simulink model "top_model_rw_desatTest"  (R2017b)
settings: Solver=FixedStepAuto  StartTime=0.0  StopTime=30000  FixedStep=.2  RelTol=1e-3  EnableMultiTasking=on
model workspace: external: MATLAB File C:\Users\Justin\Documents\00 MEng Project\PAN_ADCS\initialization\simulink_workspace_init.m (data not in the file)
undefined symbols (not defined in the file): h_init, hdmax, hmax, IAU, Imp_max, Imp_min, init, K_F, Kd, km, Kp, L_F, m_follower, match_tol, muE, ontime_max, ontime_min, q_init, s, Thrust_max, Thrust_min, wbn_init
libraries: aerolibtransform2 x12, aerolibconvert2 x8, sharedtransform x8, hEemethod x8, aerolibgravity2 x6, aerolibutil x6, aerolibcelestial x4, vrlib x4
(part 2 of 5)

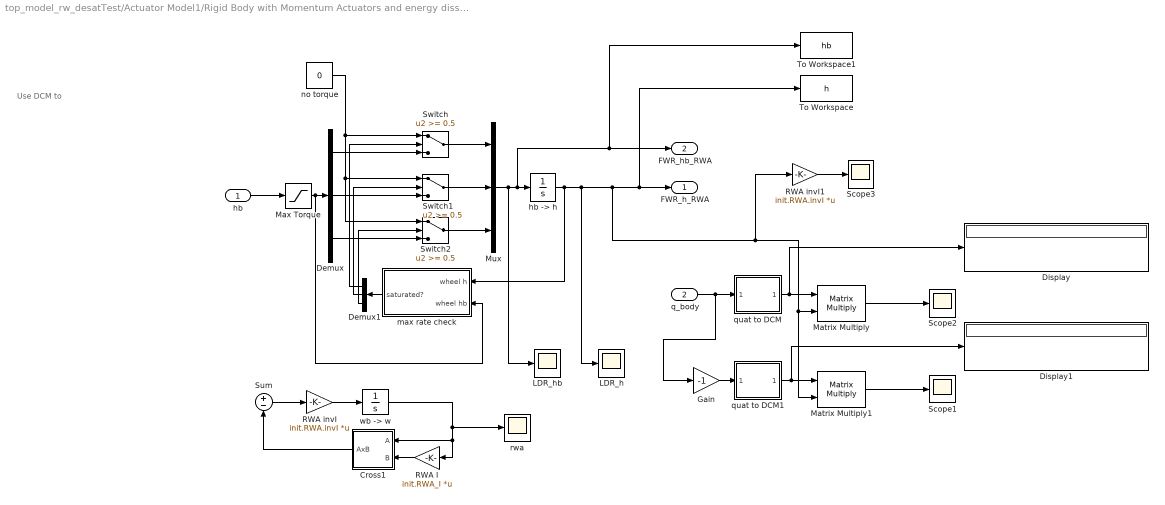
== system top_model_rw_desatTest/Actuator Model1/Rigid Body with Momentum Actuators and energy dissipation ==
  note: Use DCM to
  hb : Inport
  q_body : Inport  Port=2
  Cross1 : Subsystem
  Demux : Demux  Outputs=3
  Demux1 : Demux  Outputs=3
  Display : Display
  Display1 : Display
  Gain : Gain  Gain=-1
  LDR_h : Scope
  LDR_hb : Scope
  Matrix Multiply : Product  Multiplication=Matrix(*)
  Matrix Multiply1 : Product  Multiplication=Matrix(*)
  Max Torque : Saturate  UpperLimit=init.hdmax  LowerLimit=-init.hdmax
  Mux : Mux  Inputs=3
  RWA I : Gain  Gain=init.RWA_I  Multiplication=Matrix(K*u)
  RWA invI : Gain  Gain=init.RWA.invI  Multiplication=Matrix(K*u)
  RWA invI1 : Gain  Gain=init.RWA.invI  Multiplication=Matrix(K*u)
  Scope1 : Scope
  Scope2 : Scope
  Scope3 : Scope
  Sum : Sum  Inputs=+|-
  Switch : Switch  Threshold=0.5  SaturateOnIntegerOverflow=on  InputSameDT=on
  Switch1 : Switch  Threshold=0.5  SaturateOnIntegerOverflow=on  InputSameDT=on
  Switch2 : Switch  Threshold=0.5  SaturateOnIntegerOverflow=on  InputSameDT=on
  To Workspace : ToWorkspace  VariableName=h  SaveFormat=Timeseries  SampleTime=-1
  To Workspace1 : ToWorkspace  VariableName=hb  SaveFormat=Timeseries  SampleTime=-1
  "hb -> h" : Integrator  InitialCondition=init.FWR.h
  max rate check : Subsystem
  no torque : Constant  Value=0
  quat to DCM : Subsystem  mask(Direction Cosine Matrix){}
      mask help: Determines the 3x3 Direction Cosine Matrix (DCM) from a 4x1 quaternion orientation vector. The outputted DCM transforms vectors from inertial axes to body axes. This version corrects the fucked-up MATLAB one.
      mask Help:
      | <p>This block determines the 3x3 Direction Cosine Matrix (DCM) from a 4x1 quaternion orientation vector. The outputted DCM transforms vectors from inertial axes to body axes.  This version corrects the fucked-up MATLAB one</p>
      | 
      | <p>The block input and output contain more than one signal as described below.</p>
      | 
      | <p><H4>Block Vector Input - Quaternion</H4>
      | <ul>
      | <li>q0</li>
      | <li>q1</li>
      | <li>q2</li>
      | <li>q3</li>
      | </ul>
      | </p>
      | 
      | <p><H4>Block Matrix Output - Direction Cosine Matrix  </H4>
      |     <ul>
      |    </ul>
      |    </p>
      mask Display: disp('q to Q')
  quat to DCM1 : Subsystem  mask(Direction Cosine Matrix){}
      mask help: Determines the 3x3 Direction Cosine Matrix (DCM) from a 4x1 quaternion orientation vector. The outputted DCM transforms vectors from inertial axes to body axes. This version corrects the fucked-up MATLAB one.
      mask Help:
      | <p>This block determines the 3x3 Direction Cosine Matrix (DCM) from a 4x1 quaternion orientation vector. The outputted DCM transforms vectors from inertial axes to body axes.  This version corrects the fucked-up MATLAB one</p>
      | 
      | <p>The block input and output contain more than one signal as described below.</p>
      | 
      | <p><H4>Block Vector Input - Quaternion</H4>
      | <ul>
      | <li>q0</li>
      | <li>q1</li>
      | <li>q2</li>
      | <li>q3</li>
      | </ul>
      | </p>
      | 
      | <p><H4>Block Matrix Output - Direction Cosine Matrix  </H4>
      |     <ul>
      |    </ul>
      |    </p>
      mask Display: disp('q to Q')
  rwa : Scope
  "wb -> w" : Integrator  InitialCondition=[0;0;0]
  FWR_h_RWA : Outport
  FWR_hb_RWA : Outport  Port=2
  wires:
  hb/1 -> Max Torque/1
  Mux/1 -> To Workspace1/1, FWR_hb_RWA/1, "hb -> h"/1, LDR_hb/1
  Max Torque/1 -> Demux/1, max rate check/2(wheel hb)
  max rate check/1(saturated?) -> Demux1/1
  Demux1/1 -> Switch/2
  Demux1/2 -> Switch1/2
  Demux1/3 -> Switch2/2
  no torque/1 -> Switch/1, Switch1/1, Switch2/1
  Demux/1 -> Switch/3
  Demux/2 -> Switch1/3
  Demux/3 -> Switch2/3
  Switch/1 -> Mux/1
  Switch1/1 -> Mux/2
  Switch2/1 -> Mux/3
  q_body/1 -> Gain/1, quat to DCM/1(e0 e1 e2 e3)
  quat to DCM/1(DCM) -> Display/1, Matrix Multiply/1
  Matrix Multiply/1 -> Scope2/1
  Matrix Multiply1/1 -> Scope1/1
  quat to DCM1/1(DCM) -> Display1/1, Matrix Multiply1/1
  "hb -> h"/1 -> max rate check/1(wheel h), RWA invI1/1, Matrix Multiply1/2, Matrix Multiply/2, To Workspace/1, FWR_h_RWA/1, LDR_h/1
  Gain/1 -> quat to DCM1/1(e0 e1 e2 e3)
  RWA I/1 -> Cross1/2(B)
  "wb -> w"/1 -> rwa/1, Cross1/1(A), RWA I/1
  Cross1/1(AxB) -> Sum/2
  Sum/1 -> RWA invI/1
  RWA invI/1 -> "wb -> w"/1
  RWA invI1/1 -> Scope3/1
  ? -> Sum/1

== system top_model_rw_desatTest/Actuator Model1/torque_mt ==
  A : Inport
  B : Inport  Port=2
  Mux4 : Mux  Inputs=3
  Product{,1..5} (6 alike) : Product  SaturateOnIntegerOverflow=on  InputSameDT=on  OutDataTypeStr=Inherit: Same as first input
  Sum : Sum  Inputs=+-  SaturateOnIntegerOverflow=on  InputSameDT=on  OutDataTypeStr=Inherit: Same as first input
  Sum1 : Sum  Inputs=+-  SaturateOnIntegerOverflow=on  InputSameDT=on  OutDataTypeStr=Inherit: Same as first input
  Sum2 : Sum  Inputs=+-  SaturateOnIntegerOverflow=on  InputSameDT=on  OutDataTypeStr=Inherit: Same as first input
  demux2 : Demux  Outputs=3
  demux3 : Demux  Outputs=3
  AxB : Outport  InitialOutput=0
  wires:
  Mux4/1 -> AxB/1
  Sum2/1 -> Mux4/3
  Sum1/1 -> Mux4/2
  Sum/1 -> Mux4/1
  Product5/1 -> Sum2/2
  Product4/1 -> Sum2/1
  Product3/1 -> Sum1/2
  Product2/1 -> Sum1/1
  Product1/1 -> Sum/2
  Product/1 -> Sum/1
  demux3/1 -> Product5/2, Product2/2
  demux2/2 -> Product5/1, Product/1
  demux3/2 -> Product4/2, Product1/2
  demux2/1 -> Product4/1, Product3/1
  demux3/3 -> Product3/2, Product/2
  demux2/3 -> Product2/1, Product1/1
  B/1 -> demux3/1
  A/1 -> demux2/1

== system top_model_rw_desatTest/Attitude Determination and Desired Attitude/Attitude Determination ==
  time_elapsed : Inport
  r_cs_sensor_eci : Inport  Port=2
  r_Sun2cs_sensor_body : Inport  Port=3
  r_MagField_sensor_body : Inport  Port=4
  Generate reference vectors from Ephemeris and Magnetic Field Model : Subsystem
  Subsystem : Subsystem
  quat_body_calc : Outport
  wires:
  r_cs_sensor_eci/1 -> Generate reference vectors from Ephemeris and Magnetic Field Model/2(r_cs_sensor_eci)
  time_elapsed/1 -> Generate reference vectors from Ephemeris and Magnetic Field Model/1(time_elapsed)
  r_Sun2cs_sensor_body/1 -> Subsystem/3(r_Sun2cs_sensor_body)
  r_MagField_sensor_body/1 -> Subsystem/4(r_MagField_sensor_body)
  Generate reference vectors from Ephemeris and Magnetic Field Model/1(r_Sun2cs_ref_eci) -> Subsystem/1(r_Sun2cs_ref_eci)
  Generate reference vectors from Ephemeris and Magnetic Field Model/2(r_MagField_ref_eci) -> Subsystem/2(r_MagField_ref_eci)
  Subsystem/1(quat_body_calc) -> quat_body_calc/1

== system top_model_rw_desatTest/Attitude Determination and Desired Attitude/Cross3 ==
  A : Inport
  B : Inport  Port=2
  Mux4 : Mux  Inputs=3
  Product{,1..5} (6 alike) : Product  SaturateOnIntegerOverflow=on  InputSameDT=on  OutDataTypeStr=Inherit: Same as first input
  Sum : Sum  Inputs=+-  SaturateOnIntegerOverflow=on  InputSameDT=on  OutDataTypeStr=Inherit: Same as first input
  Sum1 : Sum  Inputs=+-  SaturateOnIntegerOverflow=on  InputSameDT=on  OutDataTypeStr=Inherit: Same as first input
  Sum2 : Sum  Inputs=+-  SaturateOnIntegerOverflow=on  InputSameDT=on  OutDataTypeStr=Inherit: Same as first input
  demux2 : Demux  Outputs=3
  demux3 : Demux  Outputs=3
  AxB : Outport  InitialOutput=0
  wires:
  A/1 -> demux2/1
  B/1 -> demux3/1
  demux2/3 -> Product1/1, Product2/1
  demux3/3 -> Product/2, Product3/2
  demux2/1 -> Product3/1, Product4/1
  demux3/2 -> Product1/2, Product4/2
  demux2/2 -> Product/1, Product5/1
  demux3/1 -> Product2/2, Product5/2
  Product/1 -> Sum/1
  Product1/1 -> Sum/2
  Product2/1 -> Sum1/1
  Product3/1 -> Sum1/2
  Product4/1 -> Sum2/1
  Product5/1 -> Sum2/2
  Sum/1 -> Mux4/1
  Sum1/1 -> Mux4/2
  Sum2/1 -> Mux4/3
  Mux4/1 -> AxB/1

== system top_model_rw_desatTest/Attitude Determination and Desired Attitude/ECEF2ECI ==
  ecef : Inport
  sec : Inport  Port=2
  Direction Cosine Matrix ECI to ECEF : aerolibtransform2/Direction Cosine Matrix ECI to ECEF  red=IAU-2000/2006  year=init.year  month=October  day=20  hour=init.hour  min=init.min  sec=init.sec  deltaT=Sec  errorflag=Error  extraparamflag=off
      settings: AttributesFormatString=%<red>  SourceProductName=Aerospace Blockset  SourceProductBaseCode=AE
  Invert 3x3 Matrix : aerolibutil/Invert  3x3 Matrix
  Product1 : Product  Multiplication=Matrix(*)
  eci : Outport
  wires:
  Direction Cosine Matrix ECI to ECEF/1 -> Invert 3x3 Matrix/1
  Product1/1 -> eci/1
  sec/1 -> Direction Cosine Matrix ECI to ECEF/1
  Invert 3x3 Matrix/1 -> Product1/1
  ecef/1 -> Product1/2

== system top_model_rw_desatTest/Attitude Determination and Desired Attitude/ECEF2ECI1 ==
  ecef : Inport
  sec : Inport  Port=2
  Direction Cosine Matrix ECI to ECEF : aerolibtransform2/Direction Cosine Matrix ECI to ECEF  red=IAU-2000/2006  year=init.year  month=October  day=20  hour=init.hour  min=init.min  sec=init.sec  deltaT=Sec  errorflag=Error  extraparamflag=off
      settings: AttributesFormatString=%<red>  SourceProductName=Aerospace Blockset  SourceProductBaseCode=AE
  Invert 3x3 Matrix : aerolibutil/Invert  3x3 Matrix
  Product1 : Product  Multiplication=Matrix(*)
  eci : Outport
  wires:
  Direction Cosine Matrix ECI to ECEF/1 -> Invert 3x3 Matrix/1
  Product1/1 -> eci/1
  sec/1 -> Direction Cosine Matrix ECI to ECEF/1
  ecef/1 -> Product1/2
  Invert 3x3 Matrix/1 -> Product1/1

== system top_model_rw_desatTest/Attitude Determination and Desired Attitude/Position and Velocity to Desired Attitude in Quat ==
  r_cs_sensor_eci : Inport
  v_cs_sensor_eci : Inport  Port=2
  CreateDCM_be : Subsystem
  Display : Display
  Display1 : Display
  MATLAB Function : MATLAB Function  TreatAsAtomicUnit=on
  Memory : Memory
  Product : Product  Multiplication=Matrix(*)
  dcm2quat : MATLAB Function  TreatAsAtomicUnit=on
  quat to DCM : Subsystem  mask(Direction Cosine Matrix){}
      mask help: Determines the 3x3 Direction Cosine Matrix (DCM) from a 4x1 quaternion orientation vector. The outputted DCM transforms vectors from inertial axes to body axes. This version corrects the fucked-up MATLAB one.
      mask Help:
      | <p>This block determines the 3x3 Direction Cosine Matrix (DCM) from a 4x1 quaternion orientation vector. The outputted DCM transforms vectors from inertial axes to body axes.  This version corrects the fucked-up MATLAB one</p>
      | 
      | <p>The block input and output contain more than one signal as described below.</p>
      | 
      | <p><H4>Block Vector Input - Quaternion</H4>
      | <ul>
      | <li>q0</li>
      | <li>q1</li>
      | <li>q2</li>
      | <li>q3</li>
      | </ul>
      | </p>
      | 
      | <p><H4>Block Matrix Output - Direction Cosine Matrix  </H4>
      |     <ul>
      |    </ul>
      |    </p>
      mask Display: disp('q to Q')
  q_des : Outport
  wires:
  r_cs_sensor_eci/1 -> CreateDCM_be/1(Position)
  v_cs_sensor_eci/1 -> CreateDCM_be/2(Velocity)
  dcm2quat/1(q) -> Memory/1
  CreateDCM_be/1(DCM_be) -> dcm2quat/1(DCM_be), MATLAB Function/1(DCM_be), Product/2, Display/1
  Memory/1 -> dcm2quat/2(q_prev)
  Product/1 -> Display1/1
  quat to DCM/1(DCM) -> Product/1
  MATLAB Function/1(q) -> q_des/1

== system top_model_rw_desatTest/Attitude Determination and Desired Attitude/norm ==
  v : Inport
  Dot Product : DotProduct  InputSameDT=on  OutDataTypeStr=Inherit: Inherit via internal rule
  Math Function : Math  Operator=sqrt  SaturateOnIntegerOverflow=on
  |v| : Outport
  wires:
  Math Function/1 -> |v|/1
  Dot Product/1 -> Math Function/1
  v/1 -> Dot Product/2, Dot Product/1

== system top_model_rw_desatTest/Attitude Determination and Desired Attitude/norm1 ==
  v : Inport
  Dot Product : DotProduct  InputSameDT=on  OutDataTypeStr=Inherit: Inherit via internal rule
  Math Function : Math  Operator=sqrt  SaturateOnIntegerOverflow=on
  |v| : Outport
  wires:
  v/1 -> Dot Product/1, Dot Product/2
  Dot Product/1 -> Math Function/1
  Math Function/1 -> |v|/1

== system top_model_rw_desatTest/Attitude Determination and Desired Attitude/normalize ==
  v : Inport
  Dot Product : DotProduct  InputSameDT=on  OutDataTypeStr=Inherit: Inherit via internal rule
  Math Function : Math  Operator=sqrt  SaturateOnIntegerOverflow=on
  Product : Product  Inputs=*/  SaturateOnIntegerOverflow=on  InputSameDT=on  OutDataTypeStr=Inherit: Same as first input
  v_hat : Outport
  wires:
  v/1 -> Dot Product/1, Dot Product/2, Product/1
  Dot Product/1 -> Math Function/1
  Math Function/1 -> Product/2
  Product/1 -> v_hat/1

== system top_model_rw_desatTest/Attitude Determination and Desired Attitude1/Attitude Determination ==
  time_elapsed : Inport
  r_cs_sensor_eci : Inport  Port=2
  r_Sun2cs_sensor_body : Inport  Port=3
  r_MagField_sensor_body : Inport  Port=4
  Generate reference vectors from Ephemeris and Magnetic Field Model : Subsystem
  Subsystem : Subsystem
  quat_body_calc : Outport
  wires:
  r_cs_sensor_eci/1 -> Generate reference vectors from Ephemeris and Magnetic Field Model/2(r_cs_sensor_eci)
  time_elapsed/1 -> Generate reference vectors from Ephemeris and Magnetic Field Model/1(time_elapsed)
  r_Sun2cs_sensor_body/1 -> Subsystem/3(r_Sun2cs_sensor_body)
  r_MagField_sensor_body/1 -> Subsystem/4(r_MagField_sensor_body)
  Generate reference vectors from Ephemeris and Magnetic Field Model/1(r_Sun2cs_ref_eci) -> Subsystem/1(r_Sun2cs_ref_eci)
  Generate reference vectors from Ephemeris and Magnetic Field Model/2(r_MagField_ref_eci) -> Subsystem/2(r_MagField_ref_eci)
  Subsystem/1(quat_body_calc) -> quat_body_calc/1

== system top_model_rw_desatTest/Attitude Determination and Desired Attitude1/Cross3 ==
  A : Inport
  B : Inport  Port=2
  Mux4 : Mux  Inputs=3
  Product{,1..5} (6 alike) : Product  SaturateOnIntegerOverflow=on  InputSameDT=on  OutDataTypeStr=Inherit: Same as first input
  Sum : Sum  Inputs=+-  SaturateOnIntegerOverflow=on  InputSameDT=on  OutDataTypeStr=Inherit: Same as first input
  Sum1 : Sum  Inputs=+-  SaturateOnIntegerOverflow=on  InputSameDT=on  OutDataTypeStr=Inherit: Same as first input
  Sum2 : Sum  Inputs=+-  SaturateOnIntegerOverflow=on  InputSameDT=on  OutDataTypeStr=Inherit: Same as first input
  demux2 : Demux  Outputs=3
  demux3 : Demux  Outputs=3
  AxB : Outport  InitialOutput=0
  wires:
  A/1 -> demux2/1
  B/1 -> demux3/1
  demux2/3 -> Product1/1, Product2/1
  demux3/3 -> Product/2, Product3/2
  demux2/1 -> Product3/1, Product4/1
  demux3/2 -> Product1/2, Product4/2
  demux2/2 -> Product/1, Product5/1
  demux3/1 -> Product2/2, Product5/2
  Product/1 -> Sum/1
  Product1/1 -> Sum/2
  Product2/1 -> Sum1/1
  Product3/1 -> Sum1/2
  Product4/1 -> Sum2/1
  Product5/1 -> Sum2/2
  Sum/1 -> Mux4/1
  Sum1/1 -> Mux4/2
  Sum2/1 -> Mux4/3
  Mux4/1 -> AxB/1

== system top_model_rw_desatTest/Attitude Determination and Desired Attitude1/ECEF2ECI ==
  ecef : Inport
  sec : Inport  Port=2
  Direction Cosine Matrix ECI to ECEF : aerolibtransform2/Direction Cosine Matrix ECI to ECEF  red=IAU-2000/2006  year=init.year  month=October  day=20  hour=init.hour  min=init.min  sec=init.sec  deltaT=Sec  errorflag=Error  extraparamflag=off
      settings: AttributesFormatString=%<red>  SourceProductName=Aerospace Blockset  SourceProductBaseCode=AE
  Invert 3x3 Matrix : aerolibutil/Invert  3x3 Matrix
  Product1 : Product  Multiplication=Matrix(*)
  eci : Outport
  wires:
  Direction Cosine Matrix ECI to ECEF/1 -> Invert 3x3 Matrix/1
  Product1/1 -> eci/1
  sec/1 -> Direction Cosine Matrix ECI to ECEF/1
  Invert 3x3 Matrix/1 -> Product1/1
  ecef/1 -> Product1/2

== system top_model_rw_desatTest/Attitude Determination and Desired Attitude1/ECEF2ECI1 ==
  ecef : Inport
  sec : Inport  Port=2
  Direction Cosine Matrix ECI to ECEF : aerolibtransform2/Direction Cosine Matrix ECI to ECEF  red=IAU-2000/2006  year=init.year  month=October  day=20  hour=init.hour  min=init.min  sec=init.sec  deltaT=Sec  errorflag=Error  extraparamflag=off
      settings: AttributesFormatString=%<red>  SourceProductName=Aerospace Blockset  SourceProductBaseCode=AE
  Invert 3x3 Matrix : aerolibutil/Invert  3x3 Matrix
  Product1 : Product  Multiplication=Matrix(*)
  eci : Outport
  wires:
  Direction Cosine Matrix ECI to ECEF/1 -> Invert 3x3 Matrix/1
  Product1/1 -> eci/1
  sec/1 -> Direction Cosine Matrix ECI to ECEF/1
  ecef/1 -> Product1/2
  Invert 3x3 Matrix/1 -> Product1/1

== system top_model_rw_desatTest/Attitude Determination and Desired Attitude1/Position and Velocity to Desired Attitude in Quat ==
  r_cs_sensor_eci : Inport
  v_cs_sensor_eci : Inport  Port=2
  CreateDCM_be : Subsystem
  Display : Display
  Display1 : Display
  MATLAB Function : MATLAB Function  TreatAsAtomicUnit=on
  Memory : Memory
  Product : Product  Multiplication=Matrix(*)
  To Workspace1 : ToWorkspace  VariableName=tr  SampleTime=-1
  To Workspace2 : ToWorkspace  VariableName=q  SampleTime=-1
  To Workspace3 : ToWorkspace  VariableName=flag  SampleTime=-1
  dcm2quat : MATLAB Function  TreatAsAtomicUnit=on
  quat to DCM : Subsystem  mask(Direction Cosine Matrix){}
      mask help: Determines the 3x3 Direction Cosine Matrix (DCM) from a 4x1 quaternion orientation vector. The outputted DCM transforms vectors from inertial axes to body axes. This version corrects the fucked-up MATLAB one.
      mask Help:
      | <p>This block determines the 3x3 Direction Cosine Matrix (DCM) from a 4x1 quaternion orientation vector. The outputted DCM transforms vectors from inertial axes to body axes.  This version corrects the fucked-up MATLAB one</p>
      | 
      | <p>The block input and output contain more than one signal as described below.</p>
      | 
      | <p><H4>Block Vector Input - Quaternion</H4>
      | <ul>
      | <li>q0</li>
      | <li>q1</li>
      | <li>q2</li>
      | <li>q3</li>
      | </ul>
      | </p>
      | 
      | <p><H4>Block Matrix Output - Direction Cosine Matrix  </H4>
      |     <ul>
      |    </ul>
      |    </p>
      mask Display: disp('q to Q')
  q_des : Outport
  wires:
  r_cs_sensor_eci/1 -> CreateDCM_be/1(Position)
  v_cs_sensor_eci/1 -> CreateDCM_be/2(Velocity)
  dcm2quat/1(q) -> Memory/1, To Workspace2/1
  CreateDCM_be/1(DCM_be) -> dcm2quat/1(DCM_be), MATLAB Function/1(DCM_be), Product/2, Display/1
  dcm2quat/2(tr) -> To Workspace1/1
  dcm2quat/3(flag) -> To Workspace3/1
  Memory/1 -> dcm2quat/2(q_prev)
  Product/1 -> Display1/1
  quat to DCM/1(DCM) -> Product/1
  MATLAB Function/1(q) -> q_des/1

== system top_model_rw_desatTest/Attitude Determination and Desired Attitude1/norm ==
  v : Inport
  Dot Product : DotProduct  InputSameDT=on  OutDataTypeStr=Inherit: Inherit via internal rule
  Math Function : Math  Operator=sqrt  SaturateOnIntegerOverflow=on
  |v| : Outport
  wires:
  Math Function/1 -> |v|/1
  Dot Product/1 -> Math Function/1
  v/1 -> Dot Product/2, Dot Product/1

== system top_model_rw_desatTest/Attitude Determination and Desired Attitude1/norm1 ==
  v : Inport
  Dot Product : DotProduct  InputSameDT=on  OutDataTypeStr=Inherit: Inherit via internal rule
  Math Function : Math  Operator=sqrt  SaturateOnIntegerOverflow=on
  |v| : Outport
  wires:
  v/1 -> Dot Product/1, Dot Product/2
  Dot Product/1 -> Math Function/1
  Math Function/1 -> |v|/1

== system top_model_rw_desatTest/Attitude Determination and Desired Attitude1/normalize ==
  v : Inport
  Dot Product : DotProduct  InputSameDT=on  OutDataTypeStr=Inherit: Inherit via internal rule
  Math Function : Math  Operator=sqrt  SaturateOnIntegerOverflow=on
  Product : Product  Inputs=*/  SaturateOnIntegerOverflow=on  InputSameDT=on  OutDataTypeStr=Inherit: Same as first input
  v_hat : Outport
  wires:
  v/1 -> Dot Product/1, Dot Product/2, Product/1
  Dot Product/1 -> Math Function/1
  Math Function/1 -> Product/2
  Product/1 -> v_hat/1

== system top_model_rw_desatTest/Controller/Free Rigid Body with Momentum Actuators2 ==
  q_ref : Inport
  w_ref : Inport  Port=2
  "torque_pert " : Inport  Port=3
  Cross : Subsystem
  Demux1 : Demux
  Derivative Gain : Gain  Gain=Kd  SaturateOnIntegerOverflow=on  OutDataTypeStr=Inherit: Same as input  ParamDataTypeStr=Inherit: Same as input
  Inertia : Gain  Gain=init.I  Multiplication=Matrix(K*u)  SaturateOnIntegerOverflow=on  OutDataTypeStr=Inherit: Same as input  ParamDataTypeStr=Inherit: Same as input
  Isc inverse : Gain  Gain=init.invI  Multiplication=Matrix(K*u)  SaturateOnIntegerOverflow=on  OutDataTypeStr=Inherit: Same as input  ParamDataTypeStr=Inherit: Same as input
  Proportional Gain : Gain  Gain=Kp  SaturateOnIntegerOverflow=on  OutDataTypeStr=Inherit: Same as input  ParamDataTypeStr=Inherit: Same as input
  Quaternion Integration : Subsystem
  RWA Saturation Model (Maxon EC 32 Flat 15W 24V) : Subsystem
  Selector q(1:3) only1 : Selector  InputPortWidth=4  IndexOptions=Index vector (dialog)  Indices=[1 2 3]  OutputSizes=1
  Sum : Sum  Inputs=+--  SaturateOnIntegerOverflow=on  InputSameDT=on  OutDataTypeStr=Inherit: Same as first input
  Sum1 : Sum  Inputs=++|
  Sum3 : Sum  Inputs=|++
  compute attitude error : Subsystem
  quat_err : Scope  NumInputPorts=4
  torque_act : Scope
  torque_cmd : Scope
  "vel_rot " : Scope
  w_error : Sum  Inputs=+-
  "wdot -> w" : Integrator  InitialCondition=wbn_init
  quat : Outport
  rate : Outport  Port=2
  wires:
  Sum/1 -> Isc inverse/1
  Isc inverse/1 -> "wdot -> w"/1
  Cross/1(AxB) -> Sum/3
  Quaternion Integration/1(q_I_Body) -> compute attitude error/1(quat), quat/1
  q_ref/1 -> compute attitude error/2(quat_cmd)
  Selector q(1:3) only1/1 -> Proportional Gain/1
  w_error/1 -> Derivative Gain/1
  w_ref/1 -> w_error/2
  "wdot -> w"/1 -> w_error/1, Inertia/1, Cross/1(A), Quaternion Integration/1(w_Body), rate/1
  Demux1/4 -> quat_err/4
  Demux1/1 -> quat_err/1
  compute attitude error/1(quat error) -> Demux1/1, Selector q(1:3) only1/1
  Demux1/2 -> quat_err/2
  Demux1/3 -> quat_err/3
  "torque_pert "/1 -> Sum/1
  Derivative Gain/1 -> Sum1/2
  Proportional Gain/1 -> Sum1/1
  Sum3/1 -> Cross/2(B)
  Inertia/1 -> Sum3/1
  RWA Saturation Model (Maxon EC 32 Flat 15W 24V)/2(h_act) -> "vel_rot "/1, Sum3/2
  Sum1/1 -> torque_cmd/1, RWA Saturation Model (Maxon EC 32 Flat 15W 24V)/1(hb_com)
  RWA Saturation Model (Maxon EC 32 Flat 15W 24V)/1(hb_act) -> Sum/2, torque_act/1

== system top_model_rw_desatTest/Controller/Normal Mode Control System ==
  note: m = k/|B| * (h-h_ref) X b
  q_cmd : Inport
  q_body : Inport  Port=2
  w_cmd : Inport  Port=3
  w_body : Inport  Port=4
  LDR_h_rw : Inport  Port=5
  LDR_mag_field_body : Inport  Port=6
  Action Port : ActionPort  PropagateVarSize=During execution  ActionType=elseif
  Constant : Constant  Value=[0;0;0]
  Constant1 : Constant  Value=init.h_des
  Cross3 : Subsystem
  Demux1 : Demux
  Derivative Gain : Gain  Gain=Kd  SaturateOnIntegerOverflow=on  OutDataTypeStr=Inherit: Same as input  ParamDataTypeStr=Inherit: Same as input
  Dot Product : DotProduct  InputSameDT=on  OutDataTypeStr=Inherit: Inherit via internal rule
  Magnet Torquer : Subsystem
  Product2 : Product  Inputs=*/
  Prop Gain1 : Gain  Gain=.001
  Proportional Gain : Gain  Gain=Kp  SaturateOnIntegerOverflow=on  OutDataTypeStr=Inherit: Same as input  ParamDataTypeStr=Inherit: Same as input
  Scope : Scope
  Scope1 : Scope
  Selector q(1:3) only1 : Selector  InputPortWidth=4  IndexOptions=Index vector (dialog)  Indices=[1 2 3]  OutputSizes=1
  Sum1 : Sum  Inputs=++|
  To Workspace : ToWorkspace  VariableName=FWR_B  SaveFormat=Timeseries  SampleTime=-1
  compute attitude error : Subsystem
  nT->T : Gain  Gain=1e-9
  quat_err : Scope  NumInputPorts=4
  w_error : Sum  Inputs=+-
  w_error1 : Sum  Inputs=-+
  hb_rw_cmd : Outport
  m_mt_cmd : Outport  Port=2
  wires:
  Proportional Gain/1 -> Sum1/1
  Derivative Gain/1 -> Sum1/2
  Demux1/2 -> quat_err/2
  w_error/1 -> Derivative Gain/1
  Demux1/3 -> quat_err/3
  Demux1/1 -> quat_err/1
  compute attitude error/1(quat error) -> Demux1/1, Selector q(1:3) only1/1
  w_body/1 -> w_error/1
  q_body/1 -> compute attitude error/1(quat)
  Demux1/4 -> quat_err/4
  q_cmd/1 -> compute attitude error/2(quat_cmd)
  Selector q(1:3) only1/1 -> Proportional Gain/1
  Sum1/1 -> hb_rw_cmd/1
  LDR_mag_field_body/1 -> nT->T/1
  Dot Product/1 -> Product2/2
  Cross3/1(AxB) -> Product2/1
  Prop Gain1/1 -> Cross3/1(A)
  LDR_h_rw/1 -> w_error1/1
  w_error1/1 -> Prop Gain1/1
  Constant1/1 -> w_error1/2
  nT->T/1 -> To Workspace/1, Dot Product/2, Dot Product/1, Cross3/2(B)
  w_cmd/1 -> w_error/2
  Product2/1 -> Scope1/1, Magnet Torquer/1(m_mt_des)
  Magnet Torquer/1(m_mt_cmd) -> Scope/1, m_mt_cmd/1

== system top_model_rw_desatTest/Controller/Propulsion ==
  Impulse_cmd_body : Inport
  pos_fire : Inport  Port=2
  pos_eci : Inport  Port=3
  Clock : Clock
  Enabled Subsystem : Subsystem  TreatAsAtomicUnit=on
  MATLAB Function : MATLAB Function  TreatAsAtomicUnit=on
  Subsystem : Subsystem
  To Workspace : ToWorkspace  VariableName=onVec  SaveFormat=Timeseries  SampleTime=-1
  To Workspace1 : ToWorkspace  VariableName=Best3  SaveFormat=Timeseries  SampleTime=-1
  To Workspace2 : ToWorkspace  VariableName=t_vector  SaveFormat=Timeseries  SampleTime=-1
  Force_applied : Outport
  wires:
  Impulse_cmd_body/1 -> MATLAB Function/1(Target)
  MATLAB Function/1(t_vector1stage) -> To Workspace2/1
  MATLAB Function/2(Best_3_names) -> To Workspace1/1
  MATLAB Function/3(onVec) -> To Workspace/1
  Enabled Subsystem/1(Out1) -> Force_applied/1

== system top_model_rw_desatTest/Controller/quat to DCM ==
  e0 e1 e2 e3 : Inport
  Demux : Demux
  Gain1 : Gain  Gain=2  SaturateOnIntegerOverflow=on  OutDataTypeStr=Inherit: Same as input  ParamDataTypeStr=Inherit: Same as input
  Gain2 : Gain  Gain=2  SaturateOnIntegerOverflow=on  OutDataTypeStr=Inherit: Same as input  ParamDataTypeStr=Inherit: Same as input
  Matrix Gain : Gain  Gain=eye(3,3)  SaturateOnIntegerOverflow=on  OutDataTypeStr=Inherit: Same as input  ParamDataTypeStr=Inherit: Same as input
  Mux : Mux  Inputs=3
  Product : Product  SaturateOnIntegerOverflow=on  InputSameDT=on  OutDataTypeStr=Inherit: Same as first input
  Product1 : Product  SaturateOnIntegerOverflow=on  InputSameDT=on  OutDataTypeStr=Inherit: Same as first input
  Subsystem : Subsystem
      mask Display: disp('3x3 cross matrix')
  Sum1 : Sum  Inputs=|+-  SaturateOnIntegerOverflow=on  InputSameDT=on  OutDataTypeStr=Inherit: Same as first input
  Sum8 : Sum  Inputs=|+-+  SaturateOnIntegerOverflow=on  InputSameDT=on  OutDataTypeStr=Inherit: Same as first input
  T1 : Math  Operator=transpose  SaturateOnIntegerOverflow=on
  T2 : Math  Operator=transpose  SaturateOnIntegerOverflow=on
  qTq : Product  Multiplication=Matrix(*)  SaturateOnIntegerOverflow=on  InputSameDT=on  OutDataTypeStr=Inherit: Same as first input
  qqT : Product  Multiplication=Matrix(*)  SaturateOnIntegerOverflow=on  InputSameDT=on  OutDataTypeStr=Inherit: Same as first input
  DCM : Outport  InitialOutput=0
  wires:
  Sum8/1 -> DCM/1
  e0 e1 e2 e3/1 -> Demux/1
  Demux/1 -> Mux/1
  Demux/2 -> Mux/2
  Demux/3 -> Mux/3
  Demux/4 -> Product/2, Product1/1, Product1/2
  Mux/1 -> T1/1, qqT/1, Subsystem/1(In1), T2/1, qTq/2
  Product/1 -> Gain1/1
  T1/1 -> qqT/2
  qqT/1 -> Gain2/1
  Gain2/1 -> Sum8/1
  Gain1/1 -> Sum8/2
  Product1/1 -> Sum1/1
  T2/1 -> qTq/1
  qTq/1 -> Sum1/2
  Sum1/1 -> Matrix Gain/1
  Matrix Gain/1 -> Sum8/3
  Subsystem/1(Out1) -> Product/1

== system top_model_rw_desatTest/Controller1/Free Rigid Body with Momentum Actuators2 ==
  q_ref : Inport
  w_ref : Inport  Port=2
  "torque_pert " : Inport  Port=3
  Cross : Subsystem
  Demux1 : Demux
  Derivative Gain : Gain  Gain=Kd  SaturateOnIntegerOverflow=on  OutDataTypeStr=Inherit: Same as input  ParamDataTypeStr=Inherit: Same as input
  Inertia : Gain  Gain=init.I  Multiplication=Matrix(K*u)  SaturateOnIntegerOverflow=on  OutDataTypeStr=Inherit: Same as input  ParamDataTypeStr=Inherit: Same as input
  Isc inverse : Gain  Gain=init.invI  Multiplication=Matrix(K*u)  SaturateOnIntegerOverflow=on  OutDataTypeStr=Inherit: Same as input  ParamDataTypeStr=Inherit: Same as input
  Proportional Gain : Gain  Gain=Kp  SaturateOnIntegerOverflow=on  OutDataTypeStr=Inherit: Same as input  ParamDataTypeStr=Inherit: Same as input
  Quaternion Integration : Subsystem
  RWA Saturation Model (Maxon EC 32 Flat 15W 24V) : Subsystem
  Selector q(1:3) only1 : Selector  InputPortWidth=4  IndexOptions=Index vector (dialog)  Indices=[1 2 3]  OutputSizes=1
  Sum : Sum  Inputs=+--  SaturateOnIntegerOverflow=on  InputSameDT=on  OutDataTypeStr=Inherit: Same as first input
  Sum1 : Sum  Inputs=++|
  Sum3 : Sum  Inputs=|++
  compute attitude error : Subsystem
  quat_err : Scope  NumInputPorts=4
  torque_act : Scope
  torque_cmd : Scope
  "vel_rot " : Scope
  w_error : Sum  Inputs=+-
  "wdot -> w" : Integrator  InitialCondition=wbn_init
  quat : Outport
  rate : Outport  Port=2
  wires:
  Sum/1 -> Isc inverse/1
  Isc inverse/1 -> "wdot -> w"/1
  Cross/1(AxB) -> Sum/3
  Quaternion Integration/1(q_I_Body) -> compute attitude error/1(quat), quat/1
  q_ref/1 -> compute attitude error/2(quat_cmd)
  Selector q(1:3) only1/1 -> Proportional Gain/1
  w_error/1 -> Derivative Gain/1
  w_ref/1 -> w_error/2
  "wdot -> w"/1 -> w_error/1, Inertia/1, Cross/1(A), Quaternion Integration/1(w_Body), rate/1
  Demux1/4 -> quat_err/4
  Demux1/1 -> quat_err/1
  compute attitude error/1(quat error) -> Demux1/1, Selector q(1:3) only1/1
  Demux1/2 -> quat_err/2
  Demux1/3 -> quat_err/3
  "torque_pert "/1 -> Sum/1
  Derivative Gain/1 -> Sum1/2
  Proportional Gain/1 -> Sum1/1
  Sum3/1 -> Cross/2(B)
  Inertia/1 -> Sum3/1
  RWA Saturation Model (Maxon EC 32 Flat 15W 24V)/2(h_act) -> "vel_rot "/1, Sum3/2
  Sum1/1 -> torque_cmd/1, RWA Saturation Model (Maxon EC 32 Flat 15W 24V)/1(hb_com)
  RWA Saturation Model (Maxon EC 32 Flat 15W 24V)/1(hb_act) -> Sum/2, torque_act/1

== system top_model_rw_desatTest/Controller1/Normal Mode Control System ==
  note: m = k/|B| * (h-h_ref) X b
  q_cmd : Inport
  q_body : Inport  Port=2
  w_cmd : Inport  Port=3
  w_body : Inport  Port=4
  LDR_h_rw : Inport  Port=5
  LDR_mag_field_body : Inport  Port=6
  Action Port : ActionPort  PropagateVarSize=During execution  ActionType=elseif
  Constant : Constant  Value=[0;0;0]
  Constant1 : Constant  Value=init.h_des
  Cross3 : Subsystem
  Demux1 : Demux
  Derivative Gain : Gain  Gain=Kd  SaturateOnIntegerOverflow=on  OutDataTypeStr=Inherit: Same as input  ParamDataTypeStr=Inherit: Same as input
  Dot Product : DotProduct  InputSameDT=on  OutDataTypeStr=Inherit: Inherit via internal rule
  Magnet Torquer : Subsystem
  Product2 : Product  Inputs=*/
  Prop Gain1 : Gain  Gain=.001
  Proportional Gain : Gain  Gain=Kp  SaturateOnIntegerOverflow=on  OutDataTypeStr=Inherit: Same as input  ParamDataTypeStr=Inherit: Same as input
  Scope : Scope
  Scope1 : Scope
  Selector q(1:3) only1 : Selector  InputPortWidth=4  IndexOptions=Index vector (dialog)  Indices=[1 2 3]  OutputSizes=1
  Sum1 : Sum  Inputs=++|
  To Workspace : ToWorkspace  VariableName=B  SaveFormat=Timeseries  SampleTime=-1
  compute attitude error : Subsystem
  nT->T : Gain  Gain=1e-9
  quat_err : Scope  NumInputPorts=4
  w_error : Sum  Inputs=+-
  w_error1 : Sum  Inputs=-+
  hb_rw_cmd : Outport
  m_mt_cmd : Outport  Port=2
  wires:
  Proportional Gain/1 -> Sum1/1
  Derivative Gain/1 -> Sum1/2
  Demux1/2 -> quat_err/2
  w_error/1 -> Derivative Gain/1
  Demux1/3 -> quat_err/3
  Demux1/1 -> quat_err/1
  compute attitude error/1(quat error) -> Demux1/1, Selector q(1:3) only1/1
  w_body/1 -> w_error/1
  q_body/1 -> compute attitude error/1(quat)
  Demux1/4 -> quat_err/4
  q_cmd/1 -> compute attitude error/2(quat_cmd)
  Selector q(1:3) only1/1 -> Proportional Gain/1
  Sum1/1 -> hb_rw_cmd/1
  LDR_mag_field_body/1 -> nT->T/1
  Dot Product/1 -> Product2/2
  Cross3/1(AxB) -> Product2/1
  Prop Gain1/1 -> Cross3/1(A)
  LDR_h_rw/1 -> w_error1/1
  w_error1/1 -> Prop Gain1/1
  Constant1/1 -> w_error1/2
  nT->T/1 -> To Workspace/1, Dot Product/2, Dot Product/1, Cross3/2(B)
  w_cmd/1 -> w_error/2
  Product2/1 -> Scope1/1, Magnet Torquer/1(m_mt_des)
  Magnet Torquer/1(m_mt_cmd) -> Scope/1, m_mt_cmd/1

== system top_model_rw_desatTest/Controller1/Propulsion ==
  Impulse_cmd_body : Inport
  trigger : Inport  Port=2
  Clock : Clock
  Enabled Subsystem : Subsystem  TreatAsAtomicUnit=on
  MATLAB Function : MATLAB Function  TreatAsAtomicUnit=on
  Subsystem : Subsystem
  Subsystem1 : Subsystem
  To Workspace : ToWorkspace  VariableName=onVec  SaveFormat=Timeseries  SampleTime=-1
  To Workspace1 : ToWorkspace  VariableName=Best3  SaveFormat=Timeseries  SampleTime=-1
  To Workspace2 : ToWorkspace  VariableName=t_vector  SaveFormat=Timeseries  SampleTime=-1
  Force_applied : Outport
  wires:
  Impulse_cmd_body/1 -> MATLAB Function/1(Target)
  MATLAB Function/1(t_vector1stage) -> To Workspace2/1
  MATLAB Function/2(Best_3_names) -> To Workspace1/1
  MATLAB Function/3(onVec) -> To Workspace/1
  Enabled Subsystem/1(Out1) -> Force_applied/1
  trigger/1 -> Subsystem1/2(overwrite trigger)

== system top_model_rw_desatTest/Controller1/norm ==
  v : Inport
  Dot Product : DotProduct  InputSameDT=on  OutDataTypeStr=Inherit: Inherit via internal rule
  Math Function : Math  Operator=sqrt  SaturateOnIntegerOverflow=on
  |v| : Outport
  wires:
  Math Function/1 -> |v|/1
  Dot Product/1 -> Math Function/1
  v/1 -> Dot Product/2, Dot Product/1

== system top_model_rw_desatTest/Controller1/quat to DCM ==
  e0 e1 e2 e3 : Inport
  Demux : Demux
  Gain1 : Gain  Gain=2  SaturateOnIntegerOverflow=on  OutDataTypeStr=Inherit: Same as input  ParamDataTypeStr=Inherit: Same as input
  Gain2 : Gain  Gain=2  SaturateOnIntegerOverflow=on  OutDataTypeStr=Inherit: Same as input  ParamDataTypeStr=Inherit: Same as input
  Matrix Gain : Gain  Gain=eye(3,3)  SaturateOnIntegerOverflow=on  OutDataTypeStr=Inherit: Same as input  ParamDataTypeStr=Inherit: Same as input
  Mux : Mux  Inputs=3
  Product : Product  SaturateOnIntegerOverflow=on  InputSameDT=on  OutDataTypeStr=Inherit: Same as first input
  Product1 : Product  SaturateOnIntegerOverflow=on  InputSameDT=on  OutDataTypeStr=Inherit: Same as first input
  Subsystem : Subsystem
      mask Display: disp('3x3 cross matrix')
  Sum1 : Sum  Inputs=|+-  SaturateOnIntegerOverflow=on  InputSameDT=on  OutDataTypeStr=Inherit: Same as first input
  Sum8 : Sum  Inputs=|+-+  SaturateOnIntegerOverflow=on  InputSameDT=on  OutDataTypeStr=Inherit: Same as first input
  T1 : Math  Operator=transpose  SaturateOnIntegerOverflow=on
  T2 : Math  Operator=transpose  SaturateOnIntegerOverflow=on
  qTq : Product  Multiplication=Matrix(*)  SaturateOnIntegerOverflow=on  InputSameDT=on  OutDataTypeStr=Inherit: Same as first input
  qqT : Product  Multiplication=Matrix(*)  SaturateOnIntegerOverflow=on  InputSameDT=on  OutDataTypeStr=Inherit: Same as first input
  DCM : Outport  InitialOutput=0
  wires:
  Sum8/1 -> DCM/1
  e0 e1 e2 e3/1 -> Demux/1
  Demux/1 -> Mux/1
  Demux/2 -> Mux/2
  Demux/3 -> Mux/3
  Demux/4 -> Product/2, Product1/1, Product1/2
  Mux/1 -> T1/1, qqT/1, Subsystem/1(In1), T2/1, qTq/2
  Product/1 -> Gain1/1
  T1/1 -> qqT/2
  qqT/1 -> Gain2/1
  Gain2/1 -> Sum8/1
  Gain1/1 -> Sum8/2
  Product1/1 -> Sum1/1
  T2/1 -> qTq/1
  qTq/1 -> Sum1/2
  Sum1/1 -> Matrix Gain/1
  Matrix Gain/1 -> Sum8/3
  Subsystem/1(Out1) -> Product/1

== system top_model_rw_desatTest/FWR_Plant/Cross ==
  A : Inport
  B : Inport  Port=2
  Mux4 : Mux  Inputs=3
  Product{,1..5} (6 alike) : Product  SaturateOnIntegerOverflow=on  InputSameDT=on  OutDataTypeStr=Inherit: Same as first input
  Sum : Sum  Inputs=+-  SaturateOnIntegerOverflow=on  InputSameDT=on  OutDataTypeStr=Inherit: Same as first input
  Sum1 : Sum  Inputs=+-  SaturateOnIntegerOverflow=on  InputSameDT=on  OutDataTypeStr=Inherit: Same as first input
  Sum2 : Sum  Inputs=+-  SaturateOnIntegerOverflow=on  InputSameDT=on  OutDataTypeStr=Inherit: Same as first input
  demux2 : Demux  Outputs=3
  demux3 : Demux  Outputs=3
  AxB : Outport  InitialOutput=0
  wires:
  Mux4/1 -> AxB/1
  Sum2/1 -> Mux4/3
  Sum1/1 -> Mux4/2
  Sum/1 -> Mux4/1
  Product5/1 -> Sum2/2
  Product4/1 -> Sum2/1
  Product3/1 -> Sum1/2
  Product2/1 -> Sum1/1
  Product1/1 -> Sum/2
  Product/1 -> Sum/1
  demux3/1 -> Product5/2, Product2/2
  demux2/2 -> Product5/1, Product/1
  demux3/2 -> Product4/2, Product1/2
  demux2/1 -> Product4/1, Product3/1
  demux3/3 -> Product3/2, Product/2
  demux2/3 -> Product2/1, Product1/1
  B/1 -> demux3/1
  A/1 -> demux2/1

== system top_model_rw_desatTest/FWR_Plant/DecimalYearIncrement ==
  note: day
  clock_sec : Inport
  Add : Sum
  Constant : Constant  Value=init.year
  Constant1 : Constant  Value=init.month
  Constant2 : Constant  Value=init.day
  Constant3 : Constant  Value=init.hour
  Constant4 : Constant  Value=init.min
  Constant5 : Constant  Value=init.min
  Divide : Product  Inputs=*/
  MATLAB Function : MATLAB Function  TreatAsAtomicUnit=on
  Product2 : Product  Inputs=*/
  day2decimalYear : Constant  Value=365
  sec2day : Constant  Value=86400
  DecimalYear : Outport
  wires:
  Product2/1 -> Divide/1
  sec2day/1 -> Product2/2
  Add/1 -> DecimalYear/1
  Constant3/1 -> MATLAB Function/4(hour)
  day2decimalYear/1 -> Divide/2
  Divide/1 -> Add/1
  MATLAB Function/1(DecimalYear) -> Add/2
  Constant1/1 -> MATLAB Function/2(month)
  Constant/1 -> MATLAB Function/1(year)
  Constant4/1 -> MATLAB Function/5(minute)
  Constant5/1 -> MATLAB Function/6(second)
  clock_sec/1 -> Product2/1
  Constant2/1 -> MATLAB Function/3(day)

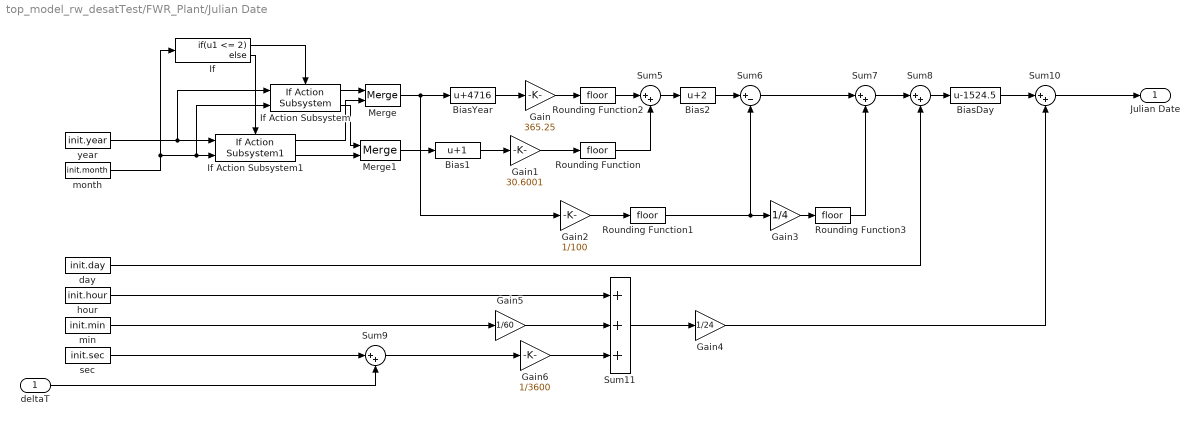
== system top_model_rw_desatTest/FWR_Plant/Julian Date ==
  deltaT : Inport  OutMin=0  PortDimensions=1
  Bias1 : Bias  Bias=1
  Bias2 : Bias  Bias=2
  BiasDay : Bias  Bias=-1524.5
  BiasYear : Bias  Bias=4716
  Gain : Gain  Gain=365.25
  Gain1 : Gain  Gain=30.6001
  Gain2 : Gain  Gain=1/100
  Gain3 : Gain  Gain=1/4
  Gain4 : Gain  Gain=1/24
  Gain5 : Gain  Gain=1/60
  Gain6 : Gain  Gain=1/3600
  If : If  IfExpression=u1 <= 2
  If Action Subsystem : aerolibconvert2/Julian Date Conversion/If Action Subsystem
      settings: SourceProductName=Aerospace Blockset  SourceProductBaseCode=AE
  If Action Subsystem1 : aerolibconvert2/Julian Date Conversion/If Action Subsystem1
      settings: SourceProductName=Aerospace Blockset  SourceProductBaseCode=AE
  Merge : Merge
  Merge1 : Merge
  Rounding Function{,1..3} (4 alike) : Rounding
  Sum{5,7..10} (5 alike) : Sum  Inputs=|++
  Sum11 : Sum  Inputs=+++
  Sum6 : Sum  Inputs=|+-
  day : Constant  Value=init.day
  hour : Constant  Value=init.hour
  min : Constant  Value=init.min
  month : Constant  Value=init.month
  sec : Constant  Value=init.sec
  year : Constant  Value=init.year
  Julian Date : Outport
  wires:
  If Action Subsystem/1 -> Merge/1
  If/2 -> If Action Subsystem1/Action
  year/1 -> If Action Subsystem/1, If Action Subsystem1/1
  If/1 -> If Action Subsystem/Action
  If Action Subsystem/2 -> Merge1/1
  Rounding Function3/1 -> Sum7/2
  deltaT/1 -> Sum9/2
  Merge1/1 -> Bias1/1
  Gain/1 -> Rounding Function2/1
  Gain2/1 -> Rounding Function1/1
  Merge/1 -> Gain2/1, BiasYear/1
  Sum9/1 -> Gain6/1
  Sum6/1 -> Sum7/1
  Gain5/1 -> Sum11/2
  BiasYear/1 -> Gain/1
  min/1 -> Gain5/1
  Gain6/1 -> Sum11/3
  Sum11/1 -> Gain4/1
  Gain3/1 -> Rounding Function3/1
  hour/1 -> Sum11/1
  If Action Subsystem1/1 -> Merge/2
  Sum7/1 -> Sum8/1
  Sum10/1 -> Julian Date/1
  day/1 -> Sum8/2
  Bias1/1 -> Gain1/1
  sec/1 -> Sum9/1
  If Action Subsystem1/2 -> Merge1/2
  Sum5/1 -> Bias2/1
  BiasDay/1 -> Sum10/1
  Gain1/1 -> Rounding Function/1
  Rounding Function1/1 -> Gain3/1, Sum6/2
  Bias2/1 -> Sum6/1
  Sum8/1 -> BiasDay/1
  Rounding Function2/1 -> Sum5/1
  Rounding Function/1 -> Sum5/2
  month/1 -> If Action Subsystem/2, If Action Subsystem1/2, If/1
  Gain4/1 -> Sum10/2

== system top_model_rw_desatTest/FWR_Plant/Quaternion Integration ==
  w_Body : Inport
  Gain : Gain  Gain=-1
  Integrator1 : Integrator  InitialCondition=init.FWR.q_init  ContinuousStateAttributes='quaternion_plant'
  Selector : Selector  InputPortWidth=4  IndexOptions=Index vector (dialog)  Indices=4  OutputSizes=1
  Switch : Switch  Criteria=u2 > Threshold
  q_normalize : Subsystem
  qderiv : Subsystem
  q_I_Body : Outport
  wires:
  qderiv/1(qd) -> Integrator1/1
  Integrator1/1 -> q_normalize/1(q_in)
  q_normalize/1(q_out) -> Gain/1, Selector/1, q_I_Body/1, Switch/1, qderiv/2(q)
  w_Body/1 -> qderiv/1(w)
  Selector/1 -> Switch/2
  Gain/1 -> Switch/3

== system top_model_rw_desatTest/FWR_Plant/norm ==
  v : Inport
  Dot Product : DotProduct  InputSameDT=on  OutDataTypeStr=Inherit: Inherit via internal rule
  Math Function : Math  Operator=sqrt  SaturateOnIntegerOverflow=on
  Saturation : Saturate  UpperLimit=1e20  LowerLimit=1e-10
  |v| : Outport
  wires:
  Saturation/1 -> |v|/1
  Math Function/1 -> Saturation/1
  Dot Product/1 -> Math Function/1
  v/1 -> Dot Product/2, Dot Product/1

== system top_model_rw_desatTest/FWR_Sensor Model/quat to DCM ==
  e0 e1 e2 e3 : Inport
  Demux : Demux
  Gain1 : Gain  Gain=2  SaturateOnIntegerOverflow=on  OutDataTypeStr=Inherit: Same as input  ParamDataTypeStr=Inherit: Same as input
  Gain2 : Gain  Gain=2  SaturateOnIntegerOverflow=on  OutDataTypeStr=Inherit: Same as input  ParamDataTypeStr=Inherit: Same as input
  Matrix Gain : Gain  Gain=eye(3,3)  SaturateOnIntegerOverflow=on  OutDataTypeStr=Inherit: Same as input  ParamDataTypeStr=Inherit: Same as input
  Mux : Mux  Inputs=3
  Product : Product  SaturateOnIntegerOverflow=on  InputSameDT=on  OutDataTypeStr=Inherit: Same as first input
  Product1 : Product  SaturateOnIntegerOverflow=on  InputSameDT=on  OutDataTypeStr=Inherit: Same as first input
  Subsystem : Subsystem
      mask Display: disp('3x3 cross matrix')
  Sum1 : Sum  Inputs=|+-  SaturateOnIntegerOverflow=on  InputSameDT=on  OutDataTypeStr=Inherit: Same as first input
  Sum8 : Sum  Inputs=|+-+  SaturateOnIntegerOverflow=on  InputSameDT=on  OutDataTypeStr=Inherit: Same as first input
  T1 : Math  Operator=transpose  SaturateOnIntegerOverflow=on
  T2 : Math  Operator=transpose  SaturateOnIntegerOverflow=on
  qTq : Product  Multiplication=Matrix(*)  SaturateOnIntegerOverflow=on  InputSameDT=on  OutDataTypeStr=Inherit: Same as first input
  qqT : Product  Multiplication=Matrix(*)  SaturateOnIntegerOverflow=on  InputSameDT=on  OutDataTypeStr=Inherit: Same as first input
  DCM : Outport  InitialOutput=0
  wires:
  Sum8/1 -> DCM/1
  e0 e1 e2 e3/1 -> Demux/1
  Demux/1 -> Mux/1
  Demux/2 -> Mux/2
  Demux/3 -> Mux/3
  Demux/4 -> Product/2, Product1/1, Product1/2
  Mux/1 -> T1/1, qqT/1, Subsystem/1(In1), T2/1, qTq/2
  Product/1 -> Gain1/1
  T1/1 -> qqT/2
  qqT/1 -> Gain2/1
  Gain2/1 -> Sum8/1
  Gain1/1 -> Sum8/2
  Product1/1 -> Sum1/1
  T2/1 -> qTq/1
  qTq/1 -> Sum1/2
  Sum1/1 -> Matrix Gain/1
  Matrix Gain/1 -> Sum8/3
  Subsystem/1(Out1) -> Product/1

== system top_model_rw_desatTest/GNC/Follower Maneuver ==
  r_follower : Inport
  v_follower : Inport  Port=2
  mu : Inport  Port=3
  x_tgt : Inport  Port=4
  m_follower : Inport  Port=5
  Imp_max : Inport  Port=6
  Imp_min : Inport  Port=7
  Update Trigger : Inport  Port=8
  Data Store Memory : DataStoreMemory  DataStoreName=man_flag  WriteAfterWriteMsg=warning  WriteAfterReadMsg=warning  ShowAdditionalParam=off
  Divide : Product  Inputs=*/
  Divide1 : Product  Inputs=**/
  Euclidean norm : hEemethod/Math Operations/Euclidean norm
      settings: SourceProductName=HEe Method Library
  Impulse Conversion : MATLAB Function  TreatAsAtomicUnit=on
  Mux1 : Mux  Inputs=3
  Optimal Latitude Calc : Subsystem
  To Workspace2 : ToWorkspace  VariableName=Thrust_vec  SaveFormat=Timeseries  SampleTime=-1
  h and E calculation : hEemethod/Math Operations/h and E calculation
      settings: SourceProductName=HEe Method Library
  long_opt : Outport
  pos_opt : Outport  Port=2
  Impulse_eci : Outport  Port=3
  ontime : Outport  Port=4
  wires:
  r_follower/1 -> h and E calculation/1, Optimal Latitude Calc/1("r ")
  h and E calculation/1 -> Mux1/1
  h and E calculation/2 -> Mux1/2
  Mux1/1 -> Optimal Latitude Calc/5(x_f)
  x_tgt/1 -> Optimal Latitude Calc/4(x_tgt)
  mu/1 -> h and E calculation/3, Optimal Latitude Calc/3(muE)
  v_follower/1 -> h and E calculation/2, Optimal Latitude Calc/2("v ")
  h and E calculation/3 -> Mux1/3
  Optimal Latitude Calc/2(long_opt) -> long_opt/1
  Optimal Latitude Calc/1(dV_opt) -> Impulse Conversion/1(dV_raw)
  Imp_min/1 -> Impulse Conversion/4(Imp_min)
  Imp_max/1 -> Impulse Conversion/3(Imp_max)
  m_follower/1 -> Impulse Conversion/2(m_follower)
  Update Trigger/1 -> Optimal Latitude Calc/6(Update Trigger)
  Optimal Latitude Calc/3(pos_opt) -> pos_opt/1
  Euclidean norm/1 -> Divide1/3, Divide/1
  Divide1/1 -> To Workspace2/1
  [Thrust_max] -> Divide/2
  Divide/1 -> Divide1/2, ontime/1
  ? -> Euclidean norm/1, Divide1/1
  Impulse Conversion/1(Imp_filt) -> Impulse_eci/1

== system top_model_rw_desatTest/GNC/Follower Orbital Elements ==
  r : Inport
  v : Inport  Port=2
  Follower True Anomaly : hEemethod/Math Operations/True Anomaly
      settings: SourceProductName=HEe Method Library
  Mux : Mux  Inputs=3
  Orbital Elements : hEemethod/Math Operations/Orbital Elements
      settings: SourceProductName=HEe Method Library
  h and E calculation : hEemethod/Math Operations/h and E calculation
      settings: SourceProductName=HEe Method Library
  a : Outport
  e : Outport  Port=2
  i : Outport  Port=3
  Ω : Outport  Port=4
  ω : Outport  Port=5
  θ : Outport  Port=6
  wires:
  h and E calculation/1 -> Mux/1
  Orbital Elements/5 -> ω/1
  Orbital Elements/2 -> e/1
  Orbital Elements/3 -> i/1
  Orbital Elements/1 -> a/1
  r/1 -> Follower True Anomaly/1, h and E calculation/1
  Orbital Elements/4 -> Ω/1
  v/1 -> Follower True Anomaly/2, h and E calculation/2
  Mux/1 -> Orbital Elements/1
  h and E calculation/2 -> Mux/2
  h and E calculation/3 -> Mux/3
  [muE] -> Follower True Anomaly/3, Orbital Elements/2, h and E calculation/3
  Follower True Anomaly/1 -> θ/1

== system top_model_rw_desatTest/GNC/Leader Orbital Elements ==
  r : Inport
  v : Inport  Port=2
  Follower True Anomaly : hEemethod/Math Operations/True Anomaly
      settings: SourceProductName=HEe Method Library
  Mux : Mux  Inputs=3
  Orbital Elements : hEemethod/Math Operations/Orbital Elements
      settings: SourceProductName=HEe Method Library
  h and E calculation : hEemethod/Math Operations/h and E calculation
      settings: SourceProductName=HEe Method Library
  a : Outport
  e : Outport  Port=2
  i : Outport  Port=3
  Ω : Outport  Port=4
  ω : Outport  Port=5
  θ : Outport  Port=6
  wires:
  h and E calculation/1 -> Mux/1
  Orbital Elements/5 -> ω/1
  Orbital Elements/2 -> e/1
  Orbital Elements/3 -> i/1
  Orbital Elements/1 -> a/1
  r/1 -> Follower True Anomaly/1, h and E calculation/1
  Orbital Elements/4 -> Ω/1
  v/1 -> Follower True Anomaly/2, h and E calculation/2
  Mux/1 -> Orbital Elements/1
  h and E calculation/2 -> Mux/2
  h and E calculation/3 -> Mux/3
  [muE] -> Follower True Anomaly/3, Orbital Elements/2, h and E calculation/3
  Follower True Anomaly/1 -> θ/1

== system top_model_rw_desatTest/GNC/Params ==
  Earth's Graviational Parameter : Constant  Value=muE
  Follower Mass : Constant  Value=m_follower
  Maximum Thrust : Constant  Value=Thrust_min
  Minimum Impulse Bit : Constant  Value=ontime_max
  Minimum Impulse Bit1 : Constant  Value=ontime_min
  Minimum Impulse Bit2 : Constant  Value=Imp_min
  Minimum Impulse Bit3 : Constant  Value=Imp_max
  Minimum Impulse Bit4 : Constant  Value=K_F
  Minimum Impulse Bit5 : Constant  Value=match_tol
  Terminator : Terminator
  Terminator1 : Terminator
  Terminator2 : Terminator
  Time for Manuever : Constant  Value=Thrust_max
  tag scope: Imp_max=global, Imp_min=global, K_F=global, Thrust_max=global, Thrust_min=global, m_f=global, match_tol=global, muE=global, ontime_max=global, ontime_min=global
  wires:
  Time for Manuever/1 -> [Thrust_max]
  Follower Mass/1 -> [m_f]
  Earth's Graviational Parameter/1 -> [muE]
  Maximum Thrust/1 -> [Thrust_min]
  Minimum Impulse Bit/1 -> [ontime_max]
  Minimum Impulse Bit1/1 -> [ontime_min]
  Minimum Impulse Bit2/1 -> [Imp_min]
  Minimum Impulse Bit3/1 -> [Imp_max]
  [Thrust_min] -> Terminator/1
  [ontime_max] -> Terminator1/1
  [ontime_min] -> Terminator2/1
  Minimum Impulse Bit4/1 -> [K_F]
  Minimum Impulse Bit5/1 -> [match_tol]

== system top_model_rw_desatTest/LDR_Plant/Cross ==
  A : Inport
  B : Inport  Port=2
  Mux4 : Mux  Inputs=3
  Product{,1..5} (6 alike) : Product  SaturateOnIntegerOverflow=on  InputSameDT=on  OutDataTypeStr=Inherit: Same as first input
  Sum : Sum  Inputs=+-  SaturateOnIntegerOverflow=on  InputSameDT=on  OutDataTypeStr=Inherit: Same as first input
  Sum1 : Sum  Inputs=+-  SaturateOnIntegerOverflow=on  InputSameDT=on  OutDataTypeStr=Inherit: Same as first input
  Sum2 : Sum  Inputs=+-  SaturateOnIntegerOverflow=on  InputSameDT=on  OutDataTypeStr=Inherit: Same as first input
  demux2 : Demux  Outputs=3
  demux3 : Demux  Outputs=3
  AxB : Outport  InitialOutput=0
  wires:
  Mux4/1 -> AxB/1
  Sum2/1 -> Mux4/3
  Sum1/1 -> Mux4/2
  Sum/1 -> Mux4/1
  Product5/1 -> Sum2/2
  Product4/1 -> Sum2/1
  Product3/1 -> Sum1/2
  Product2/1 -> Sum1/1
  Product1/1 -> Sum/2
  Product/1 -> Sum/1
  demux3/1 -> Product5/2, Product2/2
  demux2/2 -> Product5/1, Product/1
  demux3/2 -> Product4/2, Product1/2
  demux2/1 -> Product4/1, Product3/1
  demux3/3 -> Product3/2, Product/2
  demux2/3 -> Product2/1, Product1/1
  B/1 -> demux3/1
  A/1 -> demux2/1
